simulink model "Standalone_Wind_with_MPPT"  (R2024a)
settings: Solver=VariableStepAuto  StartTime=0.0  StopTime=10.0  RelTol=1e-3
libraries: spsDiodeLib x7, spsSeriesRLCBranchLib x5, spsMeanLib x2, simulink x2, spsVoltageMeasurementLib x2, spsCurrentMeasurementLib x1, spsPermanentMagnetSynchronousMachineLib x1, spsIGBTLib x1, spsThreePhaseVIMeasurementLib x1, spsWindTurbineLib x1, sps_lib x1
settings Model: Creator=91889  LastModifiedBy=91889

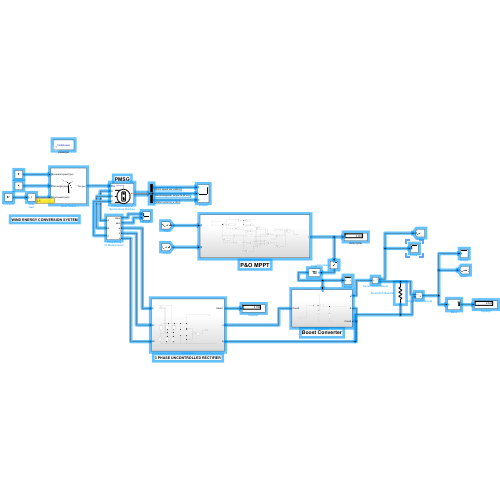
[thumbnail: Simulink's stored preview of the top-level diagram]
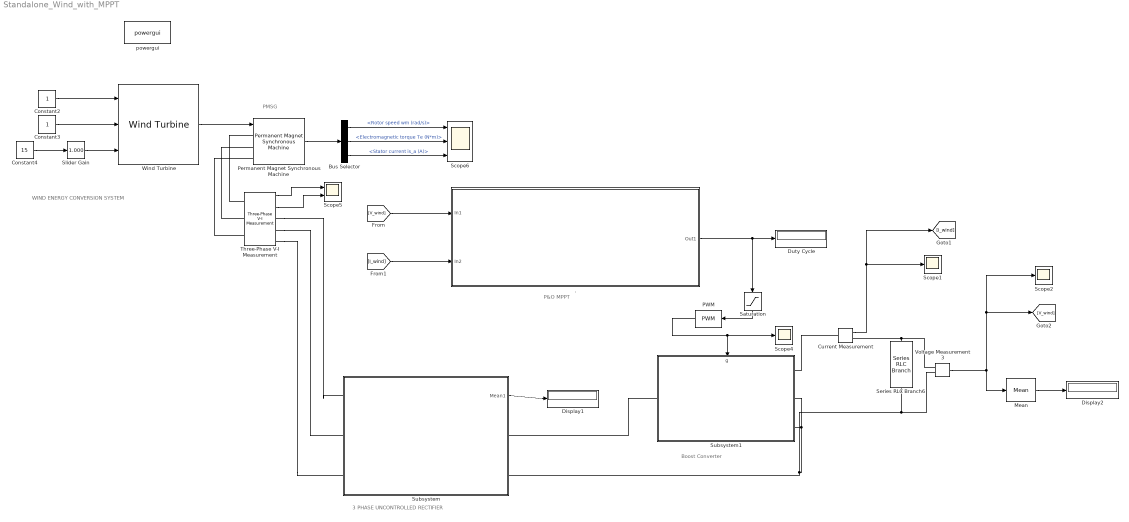
== system Standalone_Wind_with_MPPT ==
  note: Boost Converter
  note: P&O MPPT
  note: PMSG
  note: WIND ENERGY CONVERSION SYSTEM
  note: 3 PHASE UNCONTROLLED RECTIFIER
  . : Subsystem
  Bus Selector : BusSelector  OutputSignals=Rotor speed wm (rad/s),Electromagnetic torque Te (N*m),Stator current is_a (A)
  Constant2 : Constant
  Constant3 : Constant
  Constant4 : Constant  Value=15
  Current Measurement : spsCurrentMeasurementLib/Current Measurement  PhasorSimulation=off  OutputType=Complex  PSBequivalent=0
  Display1 : Display
  Display2 : Display
  Duty Cycle : Display
  Mean : spsMeanLib/Mean  Freq=60  Vinit=0  Ts=0
  PWM : simulink/Discontinuities/PWM  DisableCoverage=on  Period=50e-6  InitialDelay=0  DisallowZeroDutyCycle=off  RunAtFixedTimeIntervals=off  SampleTime=0.1
  Permanent Magnet Synchronous Machine : spsPermanentMagnetSynchronousMachineLib/Permanent Magnet Synchronous Machine  NbPhases=3  FluxDistribution=Sinusoidal  RotorType=Round  MechanicalLoad=Torque Tm  PresetModel=No  ShowDetailedParameters=on  MeasurementBus=off  Resistance=1.57  Inductance=8.5e-3  dqInductances=[8.5e-3,8.5e-3]  La=3.51e-3  MachineConstant=Flux linkage established by magnets (V.s)  Flux=0.1194  VoltageCst=151.5974  TorqueCst=1.2537  Flat=120  Mechanical=[0.0008 0.0004924 7 5e-6]  PolePairs=4  InitialConditions=[0,0, 0,0]  InitialConditions5ph=[0 0 0 0 0 0]  RefAngle=90 degrees behind phase A axis (modified Park)  IterativeDiscreteModel=Trapezoidal non iterative  TsBlock=-1  TsPowergui=0
  Saturation : Saturate  UpperLimit=0.9  LowerLimit=0.1
  Scope1 : Scope
  Scope2 : Scope
  Scope4 : Scope
  Scope5 : Scope  NumInputPorts=2
  Scope6 : Scope  NumInputPorts=3
  Series RLC Branch6 : spsSeriesRLCBranchLib/Series RLC Branch  LConnTagsString=__new0  RConnTagsString=__new0  BranchType=R  Resistance=10  Inductance=1e-3  SetiL0=off  InitialCurrent=0  Capacitance=32e-6  Setx0=off  InitialVoltage=0  Measurements=None
  Slider Gain : simulink/Math Operations/Slider Gain  gain=1.000  low=0.1  high=1
  Subsystem : Subsystem
  Subsystem1 : Subsystem
      settings: PortSchema="{\"entries\":[{\"content\":{\"sides\":[{\"content\":{\"connectorIds\":[\"LConn1\"]},\"type\":\"ConnectorPlacement.EquallySpacedRectSide\",\"uuid\":\"8b4d80fa-a07e-4510-b850-5263d03b0dea\"},{\"content\":{\"connectorIds\":[\"RConn1\",\"RConn2\",\"RConn3\"],\"side\":\"RIGHT\"},\"type\":\"ConnectorPlacement.EquallySpacedRectSide\",\"uuid\":\"d82ac879-8952-405d-86fe-c8d3c437f8a4\"},{\"content\":{\"connectorIds\":[\"In1\"],\"side\":\"TOP\"},\"type\":\"ConnectorPlacement.EquallySpacedRectSide\",\"uuid\":\"068d2ca5-aad0-402c-9038-c77e046c5036\"}]},\"type\":\"ConnectorPlacement.EquallySpacedConnector\",\"uuid\":\"75b15200-74a2-4d4a-95b9-ff3b9c90f333\"}],\"packageUris\":[\"http://schema.mathworks.com/mf0/Connector/R2020b\"],\"version\":\"1.0\"}"
  Three-Phase V-I Measurement : spsThreePhaseVIMeasurementLib/Three-Phase V-I Measurement  VoltageMeasurement=phase-to-phase  SetLabelV=off  LabelV=Vabc  Vpu=off  VpuLL=off  CurrentMeasurement=yes  SetLabelI=off  LabelI=Iabc  Ipu=off  Pbase=100e6  Vbase=500e3  OutputType=Complex  PhasorSimulation=off  PSBequivalent=0
  Voltage Measurement3 : spsVoltageMeasurementLib/Voltage Measurement  PhasorSimulation=off  OutputType=Complex  PSBequivalent=0
  Wind Turbine : spsWindTurbineLib/Wind Turbine  Pnom=1.5e6  Pelec_base=1.5e6/0.9  wind_base=12  P_wind_base=0.73  speed_nom=1.2  pitch_angle=0  c1_c6="[0.51763          116          0.4            5           21     0.006795]"  cp_nom=0.48  lambda_nom=8.1
  powergui : sps_lib/powergui  Priority=1  SimulationMode=Continuous  SampleTime=50e-6  frequency=60  Iterations=50  frequencyindice=0  Pbase=100e6  ErrMax=1e-4  UnitsV=kV  UnitsW=MW  buscounter=0  FunctionMessages=off  echomessages=off  EnableUseOfTLC=off  CurrentSourceSwitches=off  DisableSnubberDevices=off  DisableRonSwitches=off  DisableVfSwitches=off  DisplayEquations=off  AutomaticDiscreteSolvers=off  SolverType=Tustin/Backward Euler (TBE)  Interpol=off  ExternalGateDelay=off  methode=off  Ts=100  x0status=blocks  SPID=on  SwTol=0  HookPort=off  NonlinearTolerance=1e-4  nMaxIteration=100  ContinueOnMaxIteration=off  RestoreLinks=warning  ResistiveCurrentMeasurement=off  Frange=[0:2:500]  Ylog=off  Xlog=on  ShowGrid=off  save=off  variable=ZData  structure=0  ZoomFFT=off  StartTime=0.0  cycles=1  DisplayStyle=1  fundamental=60  FreqAxis=off  MaxFrequency=1000  frequencyindicesteady=1  RmsSteady=1  display=off
  wires:
  Saturation/1 -> PWM/1
  Permanent Magnet Synchronous Machine/1 -> Bus Selector/1
  Three-Phase V-I Measurement/2 -> Scope5/2
  [I_wind] -> ./2(In2)
  Wind Turbine/1 -> Permanent Magnet Synchronous Machine/1
  Slider Gain/1 -> Wind Turbine/3
  Constant4/1 -> Slider Gain/1
  Bus Selector/2 -> Scope6/2  "<Electromagnetic torque Te (N*m)>"
  Bus Selector/1 -> Scope6/1  "<Rotor speed wm (rad/s)>"
  PWM/1 -> Scope4/1, Subsystem1/1(g)
  [V_wind] -> ./1(In1)
  Bus Selector/3 -> Scope6/3  "<Stator current is_a (A)>"
  ./1(Out1) -> Duty Cycle/1, Saturation/1
  Three-Phase V-I Measurement/1 -> Scope5/1
  Constant2/1 -> Wind Turbine/1
  Constant3/1 -> Wind Turbine/2
  Voltage Measurement3/1 -> Scope2/1, [V_wind], Mean/1
  Current Measurement/1 -> [I_wind], Scope1/1
  Subsystem/1(Mean1) -> Display1/1
  Mean/1 -> Display2/1
  connections:
  Three-Phase V-I Measurement/LConn3 -- Permanent Magnet Synchronous Machine/LConn3
  Three-Phase V-I Measurement/LConn2 -- Permanent Magnet Synchronous Machine/LConn2
  Three-Phase V-I Measurement/LConn1 -- Permanent Magnet Synchronous Machine/LConn1
  Voltage Measurement3/LConn1 -- Series RLC Branch6/LConn1 -- Current Measurement/RConn1
  Three-Phase V-I Measurement/RConn1 -- Subsystem/LConn1
  Three-Phase V-I Measurement/RConn2 -- Subsystem/LConn2
  Three-Phase V-I Measurement/RConn3 -- Subsystem/LConn3
  Voltage Measurement3/LConn2 -- Subsystem/RConn2 -- Subsystem1/RConn2 -- Subsystem1/RConn3 -- Series RLC Branch6/RConn1
  Current Measurement/LConn1 -- Subsystem1/RConn1
  Subsystem1/LConn1 -- Subsystem/RConn1

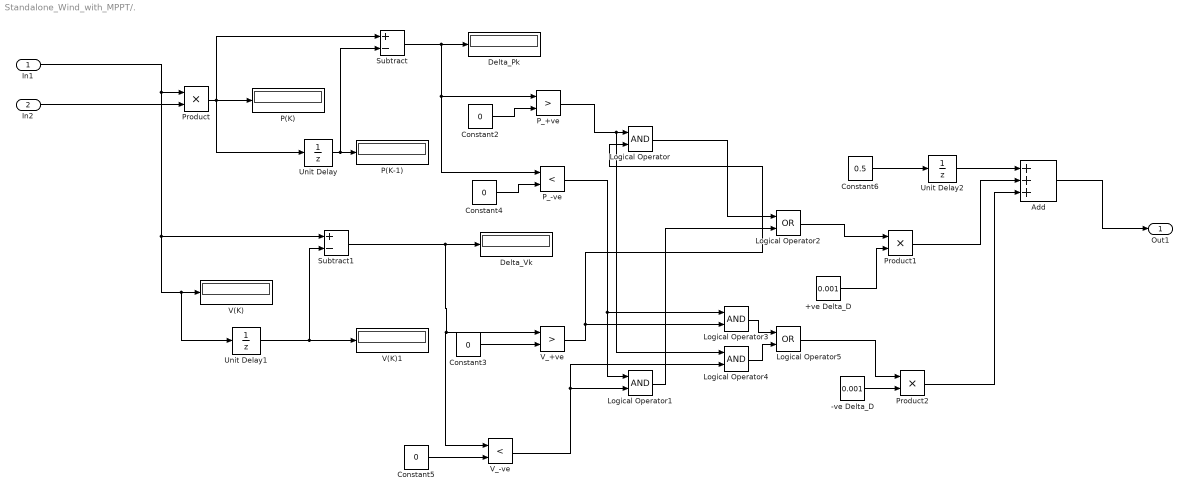
== system Standalone_Wind_with_MPPT/. ==
  In1 : Inport
  In2 : Inport  Port=2
  +ve Delta_D : Constant  Value=0.001
  -ve Delta_D : Constant  Value=0.001
  Add : Sum  Inputs=+++
  Constant{2..5} (4 alike) : Constant  Value=0
  Constant6 : Constant  Value=0.5
  Delta_Pk : Display
  Delta_Vk : Display
  Logical Operator{,1,3..4} (4 alike) : Logic  AllPortsSameDT=off  OutDataTypeStr=boolean
  Logical Operator2 : Logic  Operator=OR  AllPortsSameDT=off  OutDataTypeStr=boolean
  Logical Operator5 : Logic  Operator=OR  AllPortsSameDT=off  OutDataTypeStr=boolean
  P(K) : Display
  P(K-1) : Display
  P_+ve : RelationalOperator  Operator=>  OutDataTypeStr=boolean  RndMeth=Simplest  InputSameDT=off
  P_-ve : RelationalOperator  Operator=<  OutDataTypeStr=boolean  RndMeth=Simplest  InputSameDT=off
  Product : Product
  Product1 : Product
  Product2 : Product
  Subtract : Sum  Inputs=+-
  Subtract1 : Sum  Inputs=+-
  Unit Delay : UnitDelay  SampleTime=-1  HasFrameUpgradeWarning=on
  Unit Delay1 : UnitDelay  SampleTime=-1  HasFrameUpgradeWarning=on
  Unit Delay2 : UnitDelay  SampleTime=-1  HasFrameUpgradeWarning=on
  V(K) : Display
  V(K)1 : Display
  V_+ve : RelationalOperator  Operator=>  OutDataTypeStr=boolean  RndMeth=Simplest  InputSameDT=off
  V_-ve : RelationalOperator  Operator=<  OutDataTypeStr=boolean  RndMeth=Simplest  InputSameDT=off
  Out1 : Outport
  wires:
  Constant2/1 -> P_+ve/2
  Subtract/1 -> Delta_Pk/1, P_-ve/1, P_+ve/1
  Unit Delay1/1 -> Subtract1/2, V(K)1/1
  Product/1 -> Unit Delay/1, Subtract/1, P(K)/1
  Constant6/1 -> Unit Delay2/1
  Subtract1/1 -> V_-ve/1, V_+ve/1, Delta_Vk/1
  Logical Operator4/1 -> Logical Operator5/2
  In1/1 -> Subtract1/1, V(K)/1, Unit Delay1/1, Product/1
  Logical Operator/1 -> Logical Operator2/1
  Constant5/1 -> V_-ve/2
  Unit Delay2/1 -> Add/1
  Constant4/1 -> P_-ve/2
  Logical Operator2/1 -> Product1/1
  Logical Operator1/1 -> Logical Operator2/2
  P_-ve/1 -> Logical Operator3/1, Logical Operator1/1
  V_+ve/1 -> Logical Operator/2, Logical Operator3/2
  Logical Operator3/1 -> Logical Operator5/1
  Product1/1 -> Add/2
  Logical Operator5/1 -> Product2/1
  V_-ve/1 -> Logical Operator4/2, Logical Operator1/2
  Product2/1 -> Add/3
  Unit Delay/1 -> Subtract/2, P(K-1)/1
  P_+ve/1 -> Logical Operator4/1, Logical Operator/1
  +ve Delta_D/1 -> Product1/2
  -ve Delta_D/1 -> Product2/2
  Constant3/1 -> V_+ve/2
  Add/1 -> Out1/1
  In2/1 -> Product/2

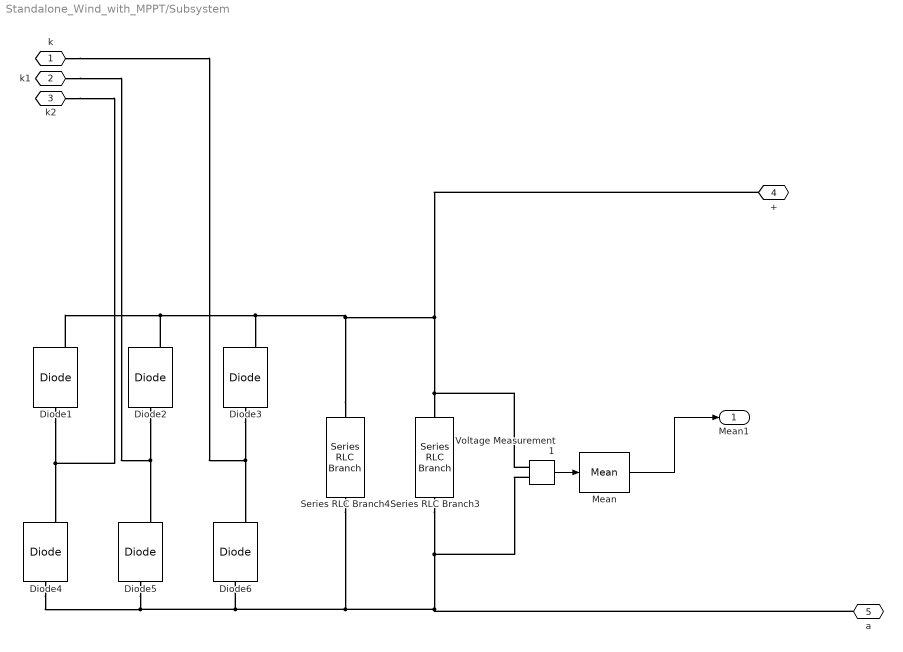
== system Standalone_Wind_with_MPPT/Subsystem ==
  Diode{1..6} (6 alike) : spsDiodeLib/Diode  Ron=0.001  Lon=0  Vf=0.8  IC=0  UseSnubber=0  Rs=500  Cs=250e-9  Measurements=on
  Mean : spsMeanLib/Mean  Freq=60  Vinit=0  Ts=0
  Series RLC Branch3 : spsSeriesRLCBranchLib/Series RLC Branch  LConnTagsString=__new0  RConnTagsString=__new0  BranchType=R  Resistance=100  Inductance=1e-3  SetiL0=off  InitialCurrent=0  Capacitance=1e-6  Setx0=off  InitialVoltage=0  Measurements=None
  Series RLC Branch4 : spsSeriesRLCBranchLib/Series RLC Branch  LConnTagsString=__new0  RConnTagsString=__new0  BranchType=C  Resistance=1  Inductance=1e-3  SetiL0=off  InitialCurrent=0  Capacitance=1e-6  Setx0=off  InitialVoltage=0  Measurements=None
  Voltage Measurement1 : spsVoltageMeasurementLib/Voltage Measurement  PhasorSimulation=off  OutputType=Complex  PSBequivalent=0
  k : PMIOPort  Side=Left
  k1 : PMIOPort  Port=2  Side=Left
  k2 : PMIOPort  Port=3  Side=Left
  + : PMIOPort  Port=4  Side=Right
  a : PMIOPort  Port=5  Side=Right
  Mean1 : Outport
  wires:
  Voltage Measurement1/1 -> Mean/1
  Mean/1 -> Mean1/1
  connections:
  Diode3/LConn1 -- k/RConn1 -- Diode6/RConn1
  Diode2/LConn1 -- k1/RConn1 -- Diode5/RConn1
  Voltage Measurement1/LConn2 -- Series RLC Branch3/RConn1 -- a/RConn1 -- Series RLC Branch4/RConn1 -- Diode6/LConn1 -- Diode5/LConn1 -- Diode4/LConn1
  Diode1/LConn1 -- k2/RConn1 -- Diode4/RConn1
  Series RLC Branch4/LConn1 -- +/RConn1 -- Voltage Measurement1/LConn1 -- Series RLC Branch3/LConn1 -- Diode3/RConn1 -- Diode1/RConn1 -- Diode2/RConn1

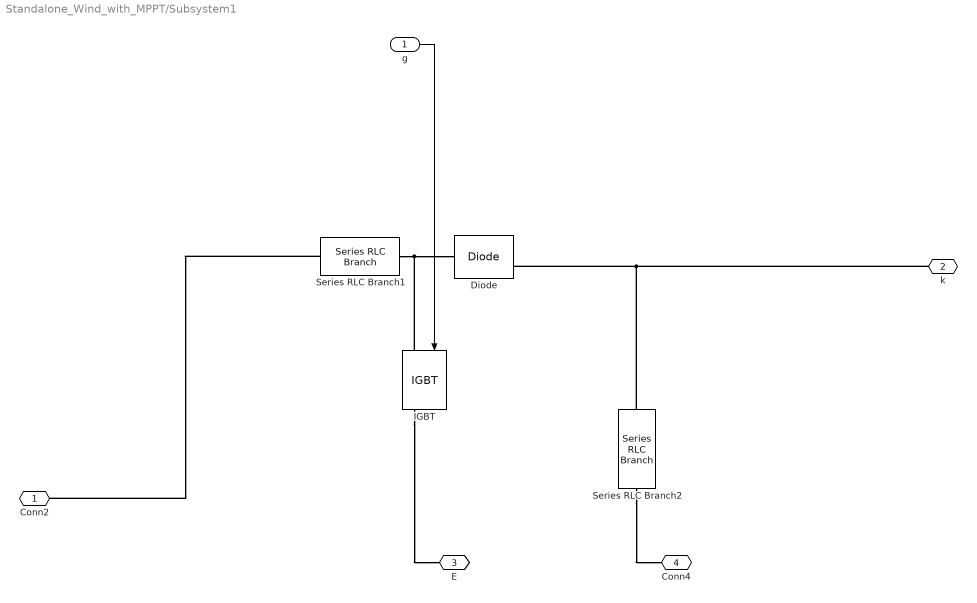
== system Standalone_Wind_with_MPPT/Subsystem1 ==
  g : Inport
  Diode : spsDiodeLib/Diode  Ron=0.001  Lon=0  Vf=0.8  IC=0  UseSnubber=0  Rs=500  Cs=250e-9  Measurements=on
  IGBT : spsIGBTLib/IGBT  Ron=0.001  Lon=0  Vf=1  Tf=1e-6  Tt=2e-6  IC=0  Rs=1e5  Cs=inf  Measurements=on
  Series RLC Branch1 : spsSeriesRLCBranchLib/Series RLC Branch  LConnTagsString=__new0  RConnTagsString=__new0  BranchType=L  Resistance=1  Inductance=5e-3  SetiL0=off  InitialCurrent=0  Capacitance=1e-6  Setx0=off  InitialVoltage=0  Measurements=None
  Series RLC Branch2 : spsSeriesRLCBranchLib/Series RLC Branch  LConnTagsString=__new0  RConnTagsString=__new0  BranchType=C  Resistance=1  Inductance=1e-3  SetiL0=off  InitialCurrent=0  Capacitance=1000e-6  Setx0=off  InitialVoltage=0  Measurements=None
  Conn2 : PMIOPort  Side=Left
  k : PMIOPort  Port=2  Side=Right
  E : PMIOPort  Port=3  Side=Right
  Conn4 : PMIOPort  Port=4  Side=Right
  wires:
  g/1 -> IGBT/1
  connections:
  Series RLC Branch1/RConn1 -- IGBT/LConn1 -- Diode/LConn1
  Series RLC Branch2/LConn1 -- k/RConn1 -- Diode/RConn1
  Series RLC Branch1/LConn1 -- Conn2/RConn1
  Series RLC Branch2/RConn1 -- Conn4/RConn1
  IGBT/RConn1 -- E/RConn1
